simulink model "test1"  (R2022b)
settings: Solver=ode4  StartTime=0.0  StopTime=20  FixedStep=0.05  RelTol=1e-3
libraries: dspsrcs4 x1, sldrtlib x1
settings Model: PacingRate=0.500000  Creator=totti  LastModifiedBy=totti

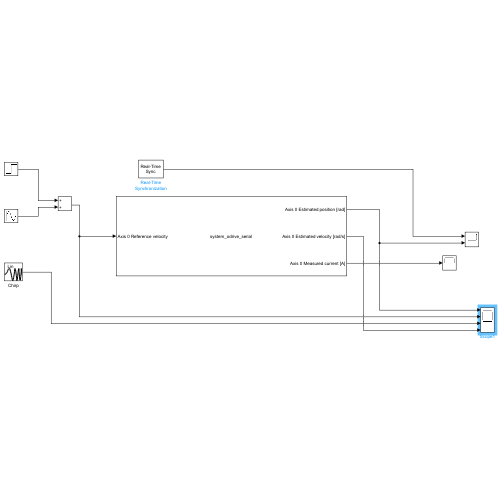
[thumbnail: Simulink's stored preview of the top-level diagram]
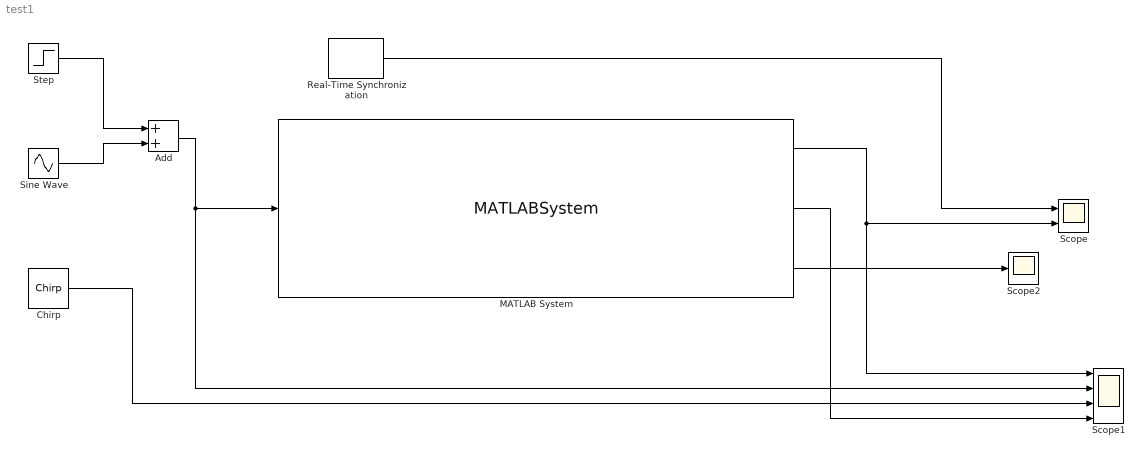
== system test1 ==
  Add : Sum
  Chirp : dspsrcs4/Chirp  sweep=Linear  mode=Unidirectional  f0=1000  f1=4000  t1=1  Tsweep=1  phase=0  Ts=0.05  spf=1  datatype=Double  OutputFrames=off
  MATLAB System : MATLABSystem  System=system_odrive_serial  Autocalibration=Disabled (fail if not calibrated)  EnableTiming=on  EnableAxis0=on  UseIndex0=off  ResetErrors0=on  ControlMode0=Velocity  VelocityLimit0=20 * pi  CurrentLimit0=40  CountsPerRotate0=8192  EnablePosition0Output=on  EnableVelocity0Output=on  EnableCurrent0Output=on  EnableError0Output=off  EnableAxis1=off  CountsPerRotate1=8192  EnablePosition1Output=off  MaxInputParameters=20  Inputs="{  }"  MaxOutputParameters=20  EnableVbusOutput=off  Outputs="{  }"
      mask Type: system_odrive_serial
      mask Display:
      | disp('system_odrive_serial');
      | port_label('input',1,'Axis 0 Reference velocity');
      | port_label('output',1,'Axis 0 Estimated position [rad]');
      | port_label('output',2,'Axis 0 Estimated velocity [rad/s]');
      | port_label('output',3,'Axis 0 Measured current [A]');
  Real-Time Synchronization : sldrtlib/Real-Time Synchronization  SampleTime=0.05  MaxMissedTicks=1000  ShowMissedTicks=on  YieldWhenWaiting=on
  Scope : Scope  NumInputPorts=2
  Scope1 : Scope  NumInputPorts=4
  Scope2 : Scope
  Sine Wave : Sin  Amplitude=5  Frequency=5  SampleTime=0
  Step : Step  Time=10  Before=-4  After=4  SampleTime=0
  wires:
  Add/1 -> Scope1/2, MATLAB System/1
  MATLAB System/1 -> Scope1/1, Scope/2
  Real-Time Synchronization/1 -> Scope/1
  MATLAB System/2 -> Scope1/4
  Sine Wave/1 -> Add/2
  Step/1 -> Add/1
  MATLAB System/3 -> Scope2/1
  Chirp/1 -> Scope1/3
